simulink model "Main_Sim_actuators_rpm"  (R2018b)
settings: Solver=FixedStepAuto  StartTime=0.0  StopTime=650  FixedStep=simParams.sample_time_s  RelTol=1e-3  EnableMultiTasking=on
libraries: actuators_lib x1, CDH_command_lib x1, Environment_lib x1, FSW_Lib x1, Sensors_Lib x1, satelliteDynamics_lib x1
settings Model: Creator=devantormey  LastModifiedBy=colem
settings OptimizationCC: LifeSpan=inf
settings DebuggingCC: SFUnexpectedBacktrackingDiag=warning  SFNoUnconditionalDefaultTransitionDiag=warning
settings SFSimCC: SimUseLocalCustomCode=off
settings RTWCC: RTWUseLocalCustomCode=off
settings CodeAppCC: StateflowObjectComments=on
settings GRTTargetCC: TargetLangStandard=C89/C90 (ANSI)  GeneratePreprocessorConditionals=Disable all
settings ConfigComp: CovMetricSettings=dw  CovHtmlReporting=on  CovSaveCumulativeToWorkspaceVar=on  CovSaveSingleToWorkspaceVar=on  CovExternalEMLEnable=off

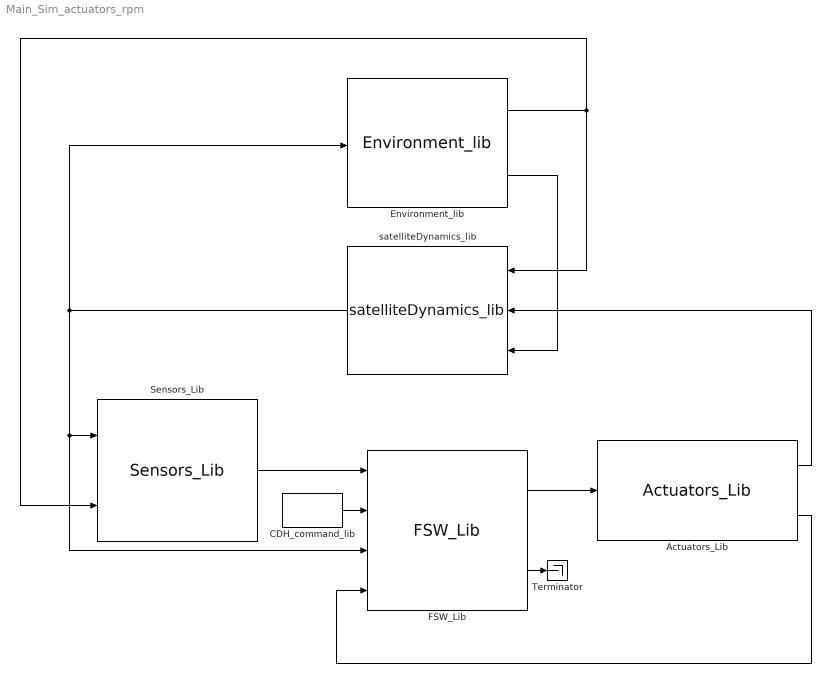
== system Main_Sim_actuators_rpm ==
  Actuators_Lib : actuators_lib/Actuators_Lib  SystemSampleTime=-1
  CDH_command_lib : CDH_command_lib/CDH_command_lib  SystemSampleTime=-1
  Environment_lib : Environment_lib/Environment_lib  SystemSampleTime=-1
  FSW_Lib : FSW_Lib/FSW_Lib  SystemSampleTime=-1
  Sensors_Lib : Sensors_Lib/Sensors_Lib  SystemSampleTime=-1
      link override Goto3: GotoTag=B_eci_T
  Terminator : Terminator
  satelliteDynamics_lib : satelliteDynamics_lib/satelliteDynamics_lib  SystemSampleTime=-1
      link override "RigidBodyDynamics/Discrete-Time Integrator ": InitialCondition=simParams.initialConditions.w0
  wires:
  FSW_Lib/1 -> Actuators_Lib/1
  Sensors_Lib/1 -> FSW_Lib/1
  satelliteDynamics_lib/1 -> Environment_lib/1, FSW_Lib/3, Sensors_Lib/1
  Environment_lib/1 -> Sensors_Lib/2, satelliteDynamics_lib/1
  Actuators_Lib/1 -> satelliteDynamics_lib/2
  FSW_Lib/2 -> Terminator/1
  CDH_command_lib/1 -> FSW_Lib/2
  Environment_lib/2 -> satelliteDynamics_lib/3
  Actuators_Lib/2 -> FSW_Lib/4
